simulink library "SimplusGT"  (R2024b)
settings: Solver=ode45  StartTime=0.0  StopTime=10.0  RelTol=1e-3
undefined symbols (not defined in the file or in its folder): ang_r, Cf, DiscIntNeverNeededParam, dspblkCoreblockFVToolHelper, gcbh, initial, Lc, Lf, m, OtherInputs, P_dc, Sbase, t0, Tm_pu, Ts, V, Vbase, w_droop, w_i, w_pll, w_tau, w_v, Wbase, wc, wfil, x0, Ybase, Zbase
libraries: spsVoltageMeasurementLib x107, spsCurrentMeasurementLib x92, spsControlledCurrentSourceLib x57, spsThreePhaseSeriesRLCBranchLib x29, spsControlledVoltageSourceLib x22, spsSeriesRLCBranchLib x15, SimplexPS_2015a x6, simulink x4, spsThreePhaseParallelRLCBranchLib x3, spsThreePhaseVIMeasurementLib x2, spsThreePhaseBreakerLib x2, $bdroot x1
(part 2 of 8)

== system SimplusGT/Complex2ReIm ==
  +- : Inport
  ->Im : Fcn  Expr=(u[1]-u[2])/2/1i
  ->Re : Fcn  Expr=(u[1]+u[2])/2
  Mux : Mux  Inputs=2
  Re Im : Outport
  wires:
  +-/1 -> ->Im/1, ->Re/1
  Mux/1 -> Re Im/1
  ->Re/1 -> Mux/1
  ->Im/1 -> Mux/2

== system SimplusGT/Conjugate ==
  note: Conjugate
      |
      | Author(s): Yitong Li
  In : Inport
  Complex to Real-Imag : ComplexToRealImag
  Gain : Gain  Gain=-1
  Real-Imag to Complex : RealImagToComplex
  Out : Outport
  wires:
  Complex to Real-Imag/1 -> Real-Imag to Complex/1
  Complex to Real-Imag/2 -> Gain/1
  Real-Imag to Complex/1 -> Out/1
  Gain/1 -> Real-Imag to Complex/2
  In/1 -> Complex to Real-Imag/1

== system SimplusGT/DC Infinite Bus (Current Type) ==
  note: Model for current-type dc infinite bus.
      |
      | Author(s): Yitong Li
  Bus Creator : BusCreator  Inputs=3
  Constant4 : Constant  Value=i
  Controlled Current Source : spsControlledCurrentSourceLib/Controlled Current Source  Initialize=on  Source_Type=AC  Amplitude=0  Phase=0  Frequency=0  Measurements=None
  Gain1 : Gain  Gain=1/Vbase
  Gain3 : Gain  Gain=Sbase/Vbase
  Product : Product
  RC : spsSeriesRLCBranchLib/Series RLC Branch  LConnTagsString=__new0  RConnTagsString=__new0  BranchType=RC  Resistance=R*V^2/Sbase  Inductance=1e-3  SetiL0=off  InitialCurrent=0  Capacitance=C/(2*pi*50)*Sbase/Vbase^2  Setx0=off  InitialVoltage=0  Measurements=None
  Voltage Measurement : spsVoltageMeasurementLib/Voltage Measurement  PhasorSimulation=off  OutputType=Complex  PSBequivalent=0
  + : PMIOPort  Side=Left
  - : PMIOPort  Port=2  Side=Left
  m : Outport
  wires:
  Constant4/1 -> [i], Gain3/1, Product/2
  [v] -> Bus Creator/1  "v"
  [i] -> Bus Creator/2  "i"
  Bus Creator/1 -> m/1
  Gain3/1 -> Controlled Current Source/1
  Gain1/1 -> Product/1, [v]
  [p] -> Bus Creator/3  "p"
  Product/1 -> [p]
  Voltage Measurement/1 -> Gain1/1
  connections:
  -/RConn1 -- RC/RConn1 -- Voltage Measurement/LConn2 -- Controlled Current Source/LConn1
  Controlled Current Source/RConn1 -- +/RConn1 -- RC/LConn1 -- Voltage Measurement/LConn1

== system SimplusGT/DC Infinite Bus (Voltage Type) ==
  note: Model for voltage-type dc infinite bus.
      |
      | Author(s): Yitong Li
  Bus Creator : BusCreator  Inputs=3
  Constant4 : Constant  Value=v
  Gain1 : Gain  Gain=Vbase
  Gain3 : Gain  Gain=1/(Sbase/Vbase)
  Product : Product
  R : spsSeriesRLCBranchLib/Series RLC Branch  LConnTagsString=__new0  RConnTagsString=__new0  BranchType=R  Resistance=R*Vbase^2/Sbase  Inductance=1e-3  SetiL0=off  InitialCurrent=0  Capacitance=1e-6  Setx0=off  InitialVoltage=0  Measurements=None
  i : spsCurrentMeasurementLib/Current Measurement  PhasorSimulation=off  OutputType=Complex  PSBequivalent=0
  v : spsControlledVoltageSourceLib/Controlled Voltage Source  Initialize=on  Source_Type=AC  Amplitude=0  Phase=0  Frequency=0  Measurements=None
  + : PMIOPort  Side=Left
  - : PMIOPort  Port=2  Side=Left
  m : Outport
  wires:
  Constant4/1 -> Product/2, [v], Gain1/1
  [v] -> Bus Creator/1  "v"
  [i] -> Bus Creator/2  "i"
  Bus Creator/1 -> m/1
  Gain1/1 -> v/1
  i/1 -> Gain3/1
  Gain3/1 -> Product/1, [i]
  [p] -> Bus Creator/3  "p"
  Product/1 -> [p]
  connections:
  v/LConn1 -- -/RConn1
  i/RConn1 -- v/RConn1
  R/RConn1 -- i/LConn1
  R/LConn1 -- +/RConn1

== system SimplusGT/DC Series RL Branch ==
  Branch1 : spsSeriesRLCBranchLib/Series RLC Branch  LConnTagsString=__new0  RConnTagsString=__new0  BranchType=RL  Resistance=Resistance/2  Inductance=Inductance/2  SetiL0=off  InitialCurrent=0  Capacitance=1e-6  Setx0=off  InitialVoltage=0  Measurements=None
  Branch2 : spsSeriesRLCBranchLib/Series RLC Branch  LConnTagsString=__new0  RConnTagsString=__new0  BranchType=RL  Resistance=Resistance/2  Inductance=Inductance/2  SetiL0=off  InitialCurrent=0  Capacitance=1e-6  Setx0=off  InitialVoltage=0  Measurements=None
  a+ : PMIOPort  Side=Left
  a- : PMIOPort  Port=2  Side=Right
  b+ : PMIOPort  Port=3  Side=Left
  b- : PMIOPort  Port=4  Side=Right
  connections:
  Branch1/RConn1 -- a-/RConn1
  Branch2/LConn1 -- b+/RConn1
  Branch2/RConn1 -- b-/RConn1
  Branch1/LConn1 -- a+/RConn1

== system SimplusGT/Discrete PI ==
  note: Digital PI controller
      |
      | Author(s): Yitong Li
  enable : Inport
  reference : Inport  Port=2
  initial : Inport  Port=3
  actual : Inport  Port=4
  Discrete-Time Integrator : DiscreteIntegrator  gainval=1  ExternalReset=rising  InitialConditionSource=external  InitialCondition=initial  SampleTime=Ts  LimitOutput=on  UpperSaturationLimit=xmax  LowerSaturationLimit=xmin  ICPrevOutput=DiscIntNeverNeededParam  ICPrevScaledInput=DiscIntNeverNeededParam
  Ierror : Sum  Inputs=+-
  Ki : Gain  Gain=Ki  SaturateOnIntegerOverflow=on  OutDataTypeStr=Inherit: Same as input  ParamDataTypeStr=Inherit: Same as input
  Kp : Gain  Gain=Kp  SaturateOnIntegerOverflow=on  OutDataTypeStr=Inherit: Same as input  ParamDataTypeStr=Inherit: Same as input
  Perror : Sum  Inputs=-+
  Product : Product  RndMeth=Zero
  Product1 : Product  RndMeth=Zero
  Saturation : Saturate  UpperLimit=xmax  LowerLimit=xmin
  Sum1 : Sum  SaturateOnIntegerOverflow=on
  Out : Outport
  wires:
  Saturation/1 -> Out/1
  Sum1/1 -> Saturation/1
  Ki/1 -> Discrete-Time Integrator/1
  Kp/1 -> Sum1/1
  Discrete-Time Integrator/1 -> Sum1/2
  enable/1 -> Discrete-Time Integrator/2, Product/2, Product1/2
  initial/1 -> Discrete-Time Integrator/3
  reference/1 -> Perror/2, Ierror/1
  actual/1 -> Ierror/2, Perror/1
  Perror/1 -> Product/1
  Product/1 -> Kp/1
  Ierror/1 -> Product1/1
  Product1/1 -> Ki/1

== system SimplusGT/Frequency Droop (iDQ -> id) ==
  note: Measurement
  note: Frequency droop controller
      |
      | Author(s): Yitong Li
      |
      | Notes:
      |
      | vq is fed into the PI controller of the PLL.
      |
      | This control assumes the input current is in DQ frame, which is the common electrical frame. It is not a practical frequency droop control which uses iabc or PQ as the input. But this controller is useful in research.
  iDQ : Inport
  wDQ : Inport  Port=2
  Constant : Constant  Value=w0
  Constant2 : Constant  Value=theta0
  Constant4 : Constant  Value=2*pi
  Constant6 : Constant  Value=i0
  Demux1 : Demux  Outputs=2
  Discrete-Time Integrator : DiscreteIntegrator  SampleTime=Ts  ICPrevOutput=DiscIntNeverNeededParam  ICPrevScaledInput=DiscIntNeverNeededParam
  Filter p : DiscreteTransferFcn  Numerator=w_tau*Ts  Denominator=[1 ((w_tau*Ts)-1)]  SampleTime=Ts
  Gain1 : Gain  Gain=1/(Sbase/Vbase)
  Gain2 : Gain  Gain=m
  Gain3 : Gain  Gain=Wbase
  Gain4 : Gain  Gain=1/Wbase
  Gain5 : Gain  Gain=1/pi
  Math Function1 : Math  Operator=mod  SignedPower=on
  Mux : Mux  Inputs=2
  Scope : Scope  NumInputPorts=4
  Sum : Sum
  Sum1 : Sum
  Sum2 : Sum  Inputs=+-
  Sum3 : Sum  Inputs=+-
  "x1y1 -> x2y2" : Subsystem  AncestorBlock=SimplusGT/x1y1 -> x2y2
      settings: LibrarySourceBlock=SimplusGT/x1y1 -> x2y2
  wdq : Outport
  theta : Outport  Port=2
  idq : Outport  Port=3
  wires:
  Gain1/1 -> Filter p/1
  Math Function1/1 -> "x1y1 -> x2y2"/2(theta), theta/1, [theta]
  Constant6/1 -> Sum2/1
  Constant/1 -> Sum/2
  [iq] -> Scope/2  "iq"
  Constant2/1 -> Sum1/2, [theta0]
  Constant4/1 -> Math Function1/2
  Gain2/1 -> Sum/1
  Sum1/1 -> Math Function1/1
  Discrete-Time Integrator/1 -> Sum1/1
  Gain5/1 -> Scope/4
  iDQ/1 -> "x1y1 -> x2y2"/1(x1y1)
  "x1y1 -> x2y2"/1(x2y2) -> idq/1, Demux1/1
  [theta0] -> Mux/1  "theta"
  Gain3/1 -> wdq/1, [w], Discrete-Time Integrator/1
  Sum2/1 -> Gain2/1
  Mux/1 -> Gain5/1  "theta"
  Demux1/1 -> Gain1/1, [id]  "id"
  [w] -> Gain4/1  "w"
  Gain4/1 -> Scope/3
  [theta] -> Mux/2  "theta"
  [id] -> Scope/1  "id"
  Filter p/1 -> Sum2/2
  Demux1/2 -> [iq]
  Sum/1 -> Sum3/1
  Sum3/1 -> Gain3/1
  wDQ/1 -> Sum3/2

== system SimplusGT/Frequency Droop (iabc -> id) ==
  note: Measurement
  note: id-frequency droop controller
      |
      | Author(s): Yitong Li
      |
      | Notes:
      |
      | The current reference should be in source convention.
      |
      | It is a id-frequency droop controller rather than a power-frequency droop controller.
  iabc : Inport
  Constant : Constant  Value=w0
  Constant2 : Constant  Value=theta0
  Constant4 : Constant  Value=2*pi
  Constant6 : Constant  Value=i0
  Demux1 : Demux  Outputs=2
  Discrete-Time Integrator : DiscreteIntegrator  SampleTime=Ts  ICPrevOutput=DiscIntNeverNeededParam  ICPrevScaledInput=DiscIntNeverNeededParam
  Filter p : DiscreteTransferFcn  Numerator=w_tau*Ts  Denominator=[1 ((w_tau*Ts)-1)]  SampleTime=Ts
  Gain1 : Gain  Gain=1/(Sbase/Vbase)
  Gain2 : Gain  Gain=m
  Gain3 : Gain  Gain=Wbase
  Gain4 : Gain  Gain=1/Wbase
  Gain5 : Gain  Gain=1/pi
  Math Function1 : Math  Operator=mod  SignedPower=on
  Mux : Mux  Inputs=2
  Scope : Scope  NumInputPorts=4
  Sum : Sum
  Sum1 : Sum
  Sum2 : Sum  Inputs=+-
  "abc -> dq (Power-Invariant)" : Subsystem  AncestorBlock=|
      | SimplusGT/abc -> dq
      | (Power-Invariant)
      settings: LibrarySourceBlock=|
      | SimplusGT/abc -> dq
      | (Power-Invariant)
  w : Outport
  theta : Outport  Port=2
  idq : Outport  Port=3
  wires:
  Sum1/1 -> Math Function1/1
  Constant2/1 -> Sum1/2, [theta0]
  Math Function1/1 -> "abc -> dq (Power-Invariant)"/2(theta), [theta], theta/1
  Gain2/1 -> Sum/1
  Discrete-Time Integrator/1 -> Sum1/1
  Filter p/1 -> Sum2/2
  Constant/1 -> Sum/2
  "abc -> dq (Power-Invariant)"/1(dq) -> idq/1, Demux1/1
  Constant4/1 -> Math Function1/2
  iabc/1 -> "abc -> dq (Power-Invariant)"/1(abc)
  Gain1/1 -> Filter p/1
  Constant6/1 -> Sum2/1
  Sum2/1 -> Gain2/1
  Sum/1 -> Gain3/1
  Gain3/1 -> [w], w/1, Discrete-Time Integrator/1
  Demux1/1 -> Gain1/1, [id]  "id"
  Gain5/1 -> Scope/4
  [iq] -> Scope/2  "iq"
  [theta0] -> Mux/1  "theta"
  [id] -> Scope/1  "id"
  Mux/1 -> Gain5/1  "theta"
  [theta] -> Mux/2  "theta"
  Demux1/2 -> [iq]
  [w] -> Gain4/1  "w"
  Gain4/1 -> Scope/3

== system SimplusGT/Frequency Droop (iabc -> id+jiq) ==
  note: Measurement
  note: Frame trabsformation
  note: Current-frequency droop controller
      |
      | Author(s): Yitong Li
      |
      | Notes:
      |
      | The current reference should be in source convention.
      |
      | This droop controller controls both d- and q-axis currents.
  iabc : Inport
  Constant : Constant  Value=id0
  Constant10 : Constant  Value=theta_d0
  Constant2 : Constant  Value=wd0
  Constant4 : Constant  Value=2*pi
  Constant5 : Constant  Value=wq0
  Constant8 : Constant  Value=iq0
  Constant9 : Constant  Value=theta_q0
  Demux1 : Demux  Outputs=2
  Discrete-Time Integrator : DiscreteIntegrator  SampleTime=Ts  ICPrevOutput=DiscIntNeverNeededParam  ICPrevScaledInput=DiscIntNeverNeededParam
  Discrete-Time Integrator1 : DiscreteIntegrator  SampleTime=Ts  ICPrevOutput=DiscIntNeverNeededParam  ICPrevScaledInput=DiscIntNeverNeededParam
  Exp : Math  SignedPower=on
  Filter p : DiscreteTransferFcn  Numerator=w_tau*Ts  Denominator=[1 ((w_tau*Ts)-1)]  SampleTime=Ts
  Filter p1 : DiscreteTransferFcn  Numerator=w_tau*Ts  Denominator=[1 ((w_tau*Ts)-1)]  SampleTime=Ts
  Gain : Gain  Gain=Wbase
  Gain1 : Gain  Gain=Wbase
  Gain2 : Gain  Gain=1/Wbase
  Gain4 : Gain  Gain=1/pi
  Gain5 : Gain  Gain=1/(Sbase/Vbase)
  Gain6 : Gain  Gain=m
  Gain7 : Gain  Gain=-1
  Gain8 : Gain  Gain=-1
  Gain9 : Gain  Gain=m
  Math Function1 : Math  Operator=mod  SignedPower=on
  Mux : Mux  Inputs=2
  Mux1 : Mux  Inputs=2
  Mux2 : Mux  Inputs=2
  Product : Product
  Scope : Scope  NumInputPorts=3
  Sum : Sum  Inputs=|+-
  Sum{1..2,4..5} (4 alike) : Sum
  Sum3 : Sum  Inputs=|+-
  "abc -> dq (Power-Invariant)1" : Subsystem  AncestorBlock=|
      | SimplusGT/abc -> dq
      | (Power-Invariant)
      settings: LibrarySourceBlock=|
      | SimplusGT/abc -> dq
      | (Power-Invariant)
  wd : Outport
  theta_d : Outport  Port=2
  wq : Outport  Port=3
  theta_q : Outport  Port=4
  wires:
  Gain2/1 -> Scope/2  "wdq"
  Discrete-Time Integrator/1 -> Sum5/1
  "abc -> dq (Power-Invariant)1"/1(dq) -> Gain5/1
  Math Function1/1 -> theta_d/1, [thetad]
  Mux2/1 -> Gain4/1  "thetadq"
  Constant5/1 -> Sum2/2
  Constant9/1 -> Sum4/2
  Gain5/1 -> Demux1/1
  Mux/1 -> Scope/1  "idq"
  Gain4/1 -> Scope/3  "thetadq"
  Demux1/2 -> [iq]
  Sum/1 -> Gain7/1
  Constant4/1 -> Math Function1/2
  Sum4/1 -> theta_q/1, [thetaq]
  Demux1/1 -> [id]
  Sum5/1 -> Math Function1/1
  Constant8/1 -> Sum3/2
  [wd] -> Mux1/1
  Constant/1 -> Sum/2
  [iq] -> Mux/2
  [thetaq] -> Mux2/2
  Mux1/1 -> Gain2/1  "wdq"
  Exp/1 -> Product/2
  [thetad] -> Mux2/1
  Constant2/1 -> Sum1/2
  [thetaq] -> Exp/1
  Constant10/1 -> Sum5/2
  [id] -> Mux/1
  Product/1 -> "abc -> dq (Power-Invariant)1"/1(abc)
  Discrete-Time Integrator1/1 -> Sum4/1
  Filter p/1 -> Sum3/1
  [thetad] -> "abc -> dq (Power-Invariant)1"/2(theta)
  [id] -> Filter p1/1
  iabc/1 -> Product/1
  [wq] -> Mux1/2
  [iq] -> Filter p/1
  Filter p1/1 -> Sum/1
  Gain9/1 -> Sum2/1
  Gain6/1 -> Sum1/1
  Gain7/1 -> Gain6/1
  Sum3/1 -> Gain8/1
  Gain8/1 -> Gain9/1
  Gain/1 -> [wd], wd/1, Discrete-Time Integrator/1
  Sum1/1 -> Gain/1
  Sum2/1 -> Gain1/1
  Gain1/1 -> [wq], wq/1, Discrete-Time Integrator1/1

== system SimplusGT/Frequency Droop (iabc -> iq) ==
  note: iq-frequency droop controller
      |
      | Author(s): Yitong Li
      |
      | Notes:
      |
      | The current reference should be in source convention.
      |
      | It is a iq-frequency droop controller rather than a power-frequency droop controller.
  note: Measurement
  iabc : Inport
  Constant : Constant  Value=w0
  Constant2 : Constant  Value=theta0
  Constant4 : Constant  Value=2*pi
  Constant6 : Constant  Value=i0
  Demux1 : Demux  Outputs=2
  Discrete-Time Integrator : DiscreteIntegrator  SampleTime=Ts  ICPrevOutput=DiscIntNeverNeededParam  ICPrevScaledInput=DiscIntNeverNeededParam
  Filter p : DiscreteTransferFcn  Numerator=w_tau*Ts  Denominator=[1 ((w_tau*Ts)-1)]  SampleTime=Ts
  Gain1 : Gain  Gain=1/(Sbase/Vbase)
  Gain2 : Gain  Gain=m
  Gain3 : Gain  Gain=Wbase
  Gain4 : Gain  Gain=1/Wbase
  Gain5 : Gain  Gain=1/pi
  Math Function1 : Math  Operator=mod  SignedPower=on
  Mux : Mux  Inputs=2
  Scope : Scope  NumInputPorts=4
  Sum : Sum
  Sum1 : Sum
  Sum2 : Sum  Inputs=+-
  "abc -> dq (Power-Invariant)1" : Subsystem  AncestorBlock=|
      | SimplusGT/abc -> dq
      | (Power-Invariant)
      settings: LibrarySourceBlock=|
      | SimplusGT/abc -> dq
      | (Power-Invariant)
  w : Outport
  theta : Outport  Port=2
  idq : Outport  Port=3
  wires:
  Demux1/2 -> Gain1/1, [iq]
  Sum1/1 -> Math Function1/1
  Gain3/1 -> Discrete-Time Integrator/1, [w], w/1
  Filter p/1 -> Sum2/2
  Constant6/1 -> Sum2/1
  Gain1/1 -> Filter p/1
  Discrete-Time Integrator/1 -> Sum1/1
  Constant2/1 -> [theta0], Sum1/2
  Sum2/1 -> Gain2/1
  Sum/1 -> Gain3/1
  Constant/1 -> Sum/2
  "abc -> dq (Power-Invariant)1"/1(dq) -> idq/1, Demux1/1
  Constant4/1 -> Math Function1/2
  Math Function1/1 -> [theta], theta/1, "abc -> dq (Power-Invariant)1"/2(theta)
  Gain2/1 -> Sum/1
  iabc/1 -> "abc -> dq (Power-Invariant)1"/1(abc)
  [iq] -> Scope/2  "iq"
  Mux/1 -> Gain5/1
  [theta0] -> Mux/1  "theta"
  [id] -> Scope/1  "id"
  Gain5/1 -> Scope/4
  [theta] -> Mux/2  "theta"
  Demux1/1 -> [id]  "id"
  Gain4/1 -> Scope/3
  [w] -> Gain4/1  "w"

== system SimplusGT/Grid-Feeding Buck (System Object) ==
  note: Matlab System Object
  note: Auxiliary
  note: Electrical Circuit
  note: Grid-feeding buck dc-dc converter.
      |
      | Author(s): Yitong Li
      |
      | Notes:
      |
      | The model is based on matlab system object.
      |
      | The model is in load convention.
  Bus Creator : BusCreator  Inputs=4
  Constant : Constant  Value=OtherInputs
  Current Measurement : spsCurrentMeasurementLib/Current Measurement  PhasorSimulation=off  OutputType=Complex  PSBequivalent=0
  Demux : Demux  Outputs=2
  Gain1 : Gain  Gain=1/Vbase
  Gain2 : Gain  Gain=Sbase/Vbase
  Gain3 : Gain  Gain=1/(Sbase/Vbase)
  MATLAB System1 : MATLABSystem  System=SimplusGT.Class.GridFeedingBuck  Ts=Ts  Para=ApparatusPara  ApparatusType=ApparatusType  PowerFlow=PowerFlow  x0=x0  DiscreMethod=DiscreMethod  LinearizationTimes=LinearizationTimes  DirectFeedthrough=DirectFeedthrough  VirtualResistor=DiscreDampingFlag  EquiInitial=true  ElecPortIOs=[1]  SimulateUsing=Code generation
      mask Type: SimplusGT.Class.GridFeedingBuck
      mask Display:
      | disp('GridFeedingBuck');
      | port_label('input',1,'u');
      | port_label('output',1,'y');
  Mux2 : Mux  Inputs=2
  Product : Product
  R_VD : spsSeriesRLCBranchLib/Series RLC Branch  LConnTagsString=__new0  RConnTagsString=__new0  BranchType=R  Resistance=DiscreDampingValue*Vbase^2/Sbase  Inductance=1e-3  SetiL0=off  InitialCurrent=0  Capacitance=1e-6  Setx0=off  InitialVoltage=0  Measurements=None
  ia : spsControlledCurrentSourceLib/Controlled Current Source  Initialize=on  Source_Type=AC  Amplitude=0  Phase=0  Frequency=0  Measurements=None
  v : spsVoltageMeasurementLib/Voltage Measurement  PhasorSimulation=off  OutputType=Complex  PSBequivalent=0
  a : PMIOPort  Side=Left
  b : PMIOPort  Port=2  Side=Left
  m : Outport
  wires:
  Gain2/1 -> ia/1
  v/1 -> Gain1/1
  [v] -> Mux2/1
  [v] -> Bus Creator/1  "v"
  Gain1/1 -> [v]
  Demux/1 -> [i]
  Mux2/1 -> MATLAB System1/1
  MATLAB System1/1 -> Demux/1
  Demux/2 -> [v_dc]
  Bus Creator/1 -> m/1
  [i] -> Gain2/1
  Product/1 -> [p]
  Constant/1 -> Mux2/2
  [v] -> Product/1  "v"
  [i_t] -> Product/2  "i"
  [i_t] -> Bus Creator/2  "i"
  [p] -> Bus Creator/3  "p"
  [v_dc] -> Bus Creator/4  "v_dc"
  Current Measurement/1 -> Gain3/1
  Gain3/1 -> [i_t]
  connections:
  b/RConn1 -- v/LConn2 -- ia/RConn1 -- R_VD/RConn1
  R_VD/LConn1 -- Current Measurement/RConn1 -- v/LConn1 -- ia/LConn1
  Current Measurement/LConn1 -- a/RConn1

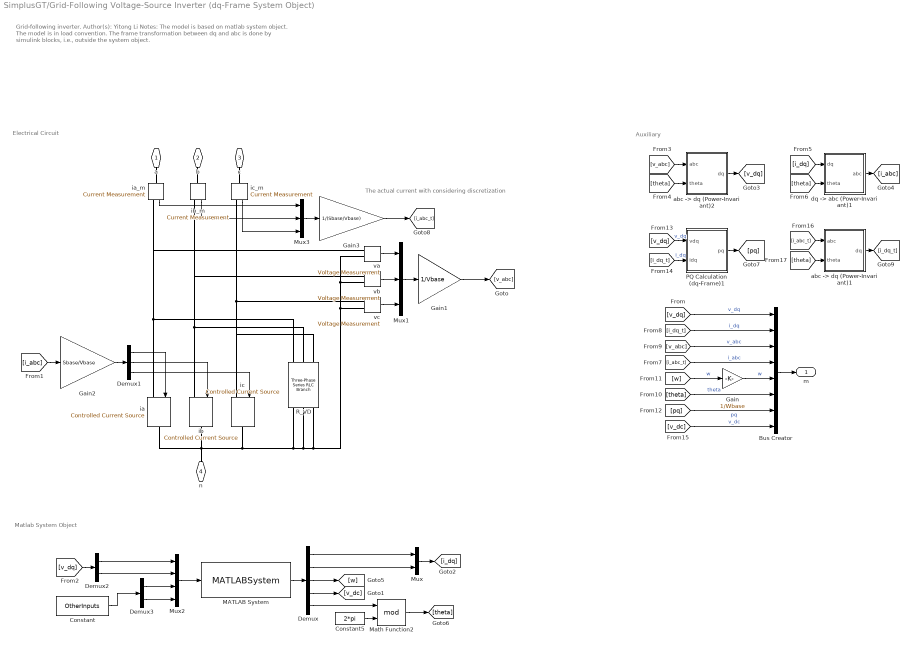
== system SimplusGT/Grid-Following Voltage-Source Inverter (dq-Frame System Object) ==
  note: Matlab System Object
  note: Auxiliary
  note: Electrical Circuit
  note: Grid-following inverter.
      |
      | Author(s): Yitong Li
      |
      | Notes:
      |
      | The model is based on matlab system object.
      |
      | The model is in load convention.
      |
      | The frame transformation between dq and abc is done by simulink blocks, i.e., outside the system object.
  note: The actual current with considering discretization
  Bus Creator : BusCreator  Inputs=8
  Constant : Constant  Value=OtherInputs
  Constant5 : Constant  Value=2*pi
  Demux : Demux  Outputs=5
  Demux1 : Demux  Outputs=3
  Demux2 : Demux  Outputs=2
  Demux3 : Demux  Outputs=2
  Gain : Gain  Gain=1/Wbase
  Gain1 : Gain  Gain=1/Vbase
  Gain2 : Gain  Gain=Sbase/Vbase
  Gain3 : Gain  Gain=1/(Sbase/Vbase)
  MATLAB System : MATLABSystem  System=SimplusGT.Class.GridFollowingVSI  Ts=Ts  Para=ApparatusPara  ApparatusType=ApparatusType  PowerFlow=PowerFlow  x0=x0  DiscreMethod=DiscreMethod  LinearizationTimes=LinearizationTimes  DirectFeedthrough=DirectFeedthrough  VirtualResistor=DiscreDampingFlag  EquiInitial=true  ElecPortIOs=[ 1, 2 ]  SimulateUsing=Code generation
      mask Type: SimplusGT.Class.GridFollowingVSI
      mask Display:
      | disp('GridFollowingVSI');
      | port_label('input',1,'u');
      | port_label('output',1,'y');
  Math Function2 : Math  Operator=mod  SignedPower=on
  Mux : Mux  Inputs=2
  Mux1 : Mux  Inputs=3
  Mux2 : Mux
  Mux3 : Mux  Inputs=3
  PQ Calculation (dq-Frame)1 : Subsystem  AncestorBlock=|
      | SimplusGT/PQ Calculation
      | (dq-Frame)
      settings: LibrarySourceBlock=|
      | SimplusGT/PQ Calculation
      | (dq-Frame)
  R_VD : spsThreePhaseSeriesRLCBranchLib/Three-Phase Series RLC Branch  LConnTagsString=A|B|C  RConnTagsString=A|B|C  BranchType=R  Resistance=DiscreDampingValue*Vbase^2/Sbase  Inductance=1e-3  Capacitance=1e-6  Measurements=None
  "abc -> dq (Power-Invariant)1" : Subsystem  AncestorBlock=|
      | SimplusGT/abc -> dq
      | (Power-Invariant)
      settings: LibrarySourceBlock=|
      | SimplusGT/abc -> dq
      | (Power-Invariant)
  "abc -> dq (Power-Invariant)2" : Subsystem  AncestorBlock=|
      | SimplusGT/abc -> dq
      | (Power-Invariant)
      settings: LibrarySourceBlock=|
      | SimplusGT/abc -> dq
      | (Power-Invariant)
  "dq -> abc (Power-Invariant)1" : Subsystem  AncestorBlock=|
      | SimplusGT/dq -> abc
      | (Power-Invariant)
      settings: LibrarySourceBlock=|
      | SimplusGT/dq -> abc
      | (Power-Invariant)
  ia : spsControlledCurrentSourceLib/Controlled Current Source  Initialize=on  Source_Type=AC  Amplitude=0  Phase=0  Frequency=0  Measurements=None
  ia_m : spsCurrentMeasurementLib/Current Measurement  PhasorSimulation=off  OutputType=Complex  PSBequivalent=0
  ib : spsControlledCurrentSourceLib/Controlled Current Source  Initialize=on  Source_Type=AC  Amplitude=0  Phase=0  Frequency=0  Measurements=None
  ib_m : spsCurrentMeasurementLib/Current Measurement  PhasorSimulation=off  OutputType=Complex  PSBequivalent=0
  ic : spsControlledCurrentSourceLib/Controlled Current Source  Initialize=on  Source_Type=AC  Amplitude=0  Phase=0  Frequency=0  Measurements=None
  ic_m : spsCurrentMeasurementLib/Current Measurement  PhasorSimulation=off  OutputType=Complex  PSBequivalent=0
  va : spsVoltageMeasurementLib/Voltage Measurement  PhasorSimulation=off  OutputType=Complex  PSBequivalent=0
  vb : spsVoltageMeasurementLib/Voltage Measurement  PhasorSimulation=off  OutputType=Complex  PSBequivalent=0
  vc : spsVoltageMeasurementLib/Voltage Measurement  PhasorSimulation=off  OutputType=Complex  PSBequivalent=0
  a : PMIOPort  Side=Left
  b : PMIOPort  Port=2  Side=Left
  c : PMIOPort  Port=3  Side=Left
  n : PMIOPort  Port=4  Side=Left
  m : Outport
  wires:
  Demux/2 -> Mux/2
  Demux/1 -> Mux/1
  Mux/1 -> [i_dq]
  Demux/3 -> [w]
  Demux1/1 -> ia/1
  Demux1/2 -> ib/1
  va/1 -> Mux1/1
  vb/1 -> Mux1/2
  Mux1/1 -> Gain1/1
  [v_dq] -> Demux2/1
  Demux2/1 -> Mux2/1
  Demux2/2 -> Mux2/2
  [v_dq] -> Bus Creator/1  "v_dq"
  [i_dq_t] -> Bus Creator/2  "i_dq"
  [v_abc] -> Bus Creator/3  "v_abc"
  [i_abc_t] -> Bus Creator/4  "i_abc"
  [theta] -> Bus Creator/6  "theta"
  [v_abc] -> "abc -> dq (Power-Invariant)2"/1(abc)
  [theta] -> "abc -> dq (Power-Invariant)2"/2(theta)
  "abc -> dq (Power-Invariant)2"/1(dq) -> [v_dq]
  [i_dq] -> "dq -> abc (Power-Invariant)1"/1(dq)
  [theta] -> "dq -> abc (Power-Invariant)1"/2(theta)
  "dq -> abc (Power-Invariant)1"/1(abc) -> [i_abc]
  Mux2/1 -> MATLAB System/1
  MATLAB System/1 -> Demux/1
  vc/1 -> Mux1/3
  Demux1/3 -> ic/1
  Demux/5 -> Math Function2/1
  Constant5/1 -> Math Function2/2
  Math Function2/1 -> [theta]
  Demux/4 -> [v_dc]
  Bus Creator/1 -> m/1
  Demux3/1 -> Mux2/3
  Demux3/2 -> Mux2/4
  Constant/1 -> Demux3/1
  [w] -> Gain/1  "w"
  Gain/1 -> Bus Creator/5  "w"
  [i_abc] -> Gain2/1
  [pq] -> Bus Creator/7  "pq"
  [v_dq] -> PQ Calculation (dq-Frame)1/1(vdq)  "v_dq"
  [i_dq_t] -> PQ Calculation (dq-Frame)1/2(idq)  "i_dq"
  PQ Calculation (dq-Frame)1/1(pq) -> [pq]
  Gain2/1 -> Demux1/1
  Gain1/1 -> [v_abc]
  [v_dc] -> Bus Creator/8  "v_dc"
  ic_m/1 -> Mux3/3
  Gain3/1 -> [i_abc_t]
  Mux3/1 -> Gain3/1
  ib_m/1 -> Mux3/2
  ia_m/1 -> Mux3/1
  [theta] -> "abc -> dq (Power-Invariant)1"/2(theta)
  [i_abc_t] -> "abc -> dq (Power-Invariant)1"/1(abc)
  "abc -> dq (Power-Invariant)1"/1(dq) -> [i_dq_t]
  connections:
  vb/LConn2 -- va/LConn2 -- vc/LConn2 -- R_VD/RConn3 -- R_VD/RConn2 -- R_VD/RConn1 -- ic/RConn1 -- ia/RConn1 -- ib/RConn1 -- n/RConn1
  R_VD/LConn1 -- va/LConn1 -- ia_m/RConn1 -- ia/LConn1
  R_VD/LConn2 -- ib_m/RConn1 -- vb/LConn1 -- ib/LConn1
  R_VD/LConn3 -- ic/LConn1 -- ic_m/RConn1 -- vc/LConn1
  ic_m/LConn1 -- c/RConn1
  ib_m/LConn1 -- b/RConn1
  ia_m/LConn1 -- a/RConn1

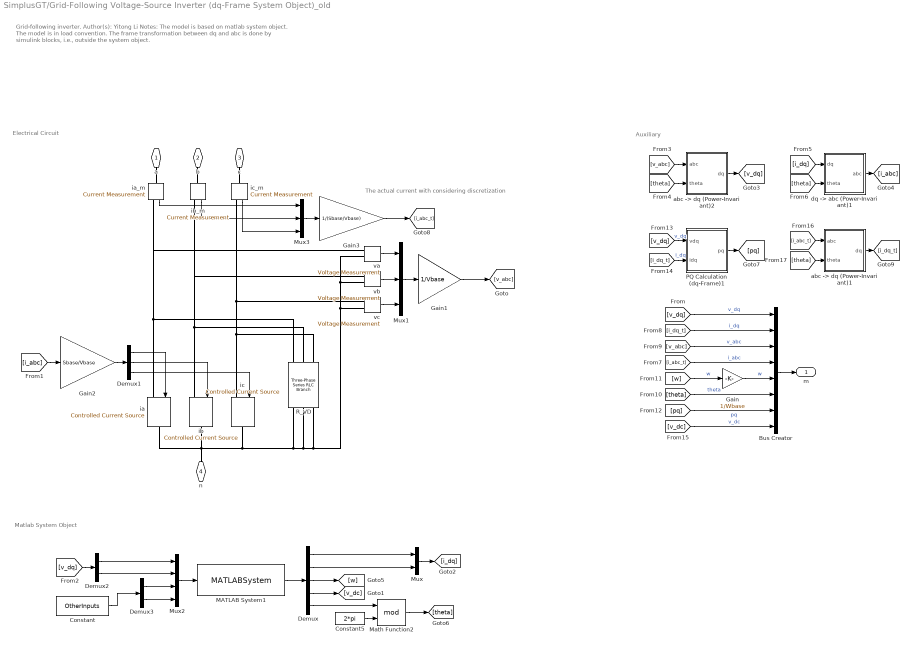
== system SimplusGT/Grid-Following Voltage-Source Inverter (dq-Frame System Object)_old ==
  note: Matlab System Object
  note: Auxiliary
  note: Electrical Circuit
  note: Grid-following inverter.
      |
      | Author(s): Yitong Li
      |
      | Notes:
      |
      | The model is based on matlab system object.
      |
      | The model is in load convention.
      |
      | The frame transformation between dq and abc is done by simulink blocks, i.e., outside the system object.
  note: The actual current with considering discretization
  Bus Creator : BusCreator  Inputs=8
  Constant : Constant  Value=OtherInputs
  Constant5 : Constant  Value=2*pi
  Demux : Demux  Outputs=5
  Demux1 : Demux  Outputs=3
  Demux2 : Demux  Outputs=2
  Demux3 : Demux  Outputs=2
  Gain : Gain  Gain=1/Wbase
  Gain1 : Gain  Gain=1/Vbase
  Gain2 : Gain  Gain=Sbase/Vbase
  Gain3 : Gain  Gain=1/(Sbase/Vbase)
  MATLAB System1 : MATLABSystem  System=SimplusGT.Class.GridFollowingVSI_old  Ts=Ts  Para=ApparatusPara  ApparatusType=ApparatusType  PowerFlow=PowerFlow  x0=x0  DiscreMethod=DiscreMethod  LinearizationTimes=LinearizationTimes  DirectFeedthrough=DirectFeedthrough  VirtualResistor=DiscreDampingFlag  EquiInitial=true  ElecPortIOs=[ 1, 2 ]  SimulateUsing=Code generation
      mask Type: SimplusGT.Class.GridFollowingVSI_old
      mask Display:
      | disp('GridFollowingVSI_old');
      | port_label('input',1,'u');
      | port_label('output',1,'y');
  Math Function2 : Math  Operator=mod  SignedPower=on
  Mux : Mux  Inputs=2
  Mux1 : Mux  Inputs=3
  Mux2 : Mux
  Mux3 : Mux  Inputs=3
  PQ Calculation (dq-Frame)1 : Subsystem  AncestorBlock=|
      | SimplusGT/PQ Calculation
      | (dq-Frame)
      settings: LibrarySourceBlock=|
      | SimplusGT/PQ Calculation
      | (dq-Frame)
  R_VD : spsThreePhaseSeriesRLCBranchLib/Three-Phase Series RLC Branch  LConnTagsString=A|B|C  RConnTagsString=A|B|C  BranchType=R  Resistance=DiscreDampingValue*Vbase^2/Sbase  Inductance=1e-3  Capacitance=1e-6  Measurements=None
  "abc -> dq (Power-Invariant)1" : Subsystem  AncestorBlock=|
      | SimplusGT/abc -> dq
      | (Power-Invariant)
      settings: LibrarySourceBlock=|
      | SimplusGT/abc -> dq
      | (Power-Invariant)
  "abc -> dq (Power-Invariant)2" : Subsystem  AncestorBlock=|
      | SimplusGT/abc -> dq
      | (Power-Invariant)
      settings: LibrarySourceBlock=|
      | SimplusGT/abc -> dq
      | (Power-Invariant)
  "dq -> abc (Power-Invariant)1" : Subsystem  AncestorBlock=|
      | SimplusGT/dq -> abc
      | (Power-Invariant)
      settings: LibrarySourceBlock=|
      | SimplusGT/dq -> abc
      | (Power-Invariant)
  ia : spsControlledCurrentSourceLib/Controlled Current Source  Initialize=on  Source_Type=AC  Amplitude=0  Phase=0  Frequency=0  Measurements=None
  ia_m : spsCurrentMeasurementLib/Current Measurement  PhasorSimulation=off  OutputType=Complex  PSBequivalent=0
  ib : spsControlledCurrentSourceLib/Controlled Current Source  Initialize=on  Source_Type=AC  Amplitude=0  Phase=0  Frequency=0  Measurements=None
  ib_m : spsCurrentMeasurementLib/Current Measurement  PhasorSimulation=off  OutputType=Complex  PSBequivalent=0
  ic : spsControlledCurrentSourceLib/Controlled Current Source  Initialize=on  Source_Type=AC  Amplitude=0  Phase=0  Frequency=0  Measurements=None
  ic_m : spsCurrentMeasurementLib/Current Measurement  PhasorSimulation=off  OutputType=Complex  PSBequivalent=0
  va : spsVoltageMeasurementLib/Voltage Measurement  PhasorSimulation=off  OutputType=Complex  PSBequivalent=0
  vb : spsVoltageMeasurementLib/Voltage Measurement  PhasorSimulation=off  OutputType=Complex  PSBequivalent=0
  vc : spsVoltageMeasurementLib/Voltage Measurement  PhasorSimulation=off  OutputType=Complex  PSBequivalent=0
  a : PMIOPort  Side=Left
  b : PMIOPort  Port=2  Side=Left
  c : PMIOPort  Port=3  Side=Left
  n : PMIOPort  Port=4  Side=Left
  m : Outport
  wires:
  Demux/2 -> Mux/2
  Demux/1 -> Mux/1
  Mux/1 -> [i_dq]
  Demux/3 -> [w]
  Demux1/1 -> ia/1
  Demux1/2 -> ib/1
  va/1 -> Mux1/1
  vb/1 -> Mux1/2
  Mux1/1 -> Gain1/1
  [v_dq] -> Demux2/1
  Demux2/1 -> Mux2/1
  Demux2/2 -> Mux2/2
  [v_dq] -> Bus Creator/1  "v_dq"
  [i_dq_t] -> Bus Creator/2  "i_dq"
  [v_abc] -> Bus Creator/3  "v_abc"
  [i_abc_t] -> Bus Creator/4  "i_abc"
  [theta] -> Bus Creator/6  "theta"
  [v_abc] -> "abc -> dq (Power-Invariant)2"/1(abc)
  [theta] -> "abc -> dq (Power-Invariant)2"/2(theta)
  "abc -> dq (Power-Invariant)2"/1(dq) -> [v_dq]
  [i_dq] -> "dq -> abc (Power-Invariant)1"/1(dq)
  [theta] -> "dq -> abc (Power-Invariant)1"/2(theta)
  "dq -> abc (Power-Invariant)1"/1(abc) -> [i_abc]
  Mux2/1 -> MATLAB System1/1
  MATLAB System1/1 -> Demux/1
  vc/1 -> Mux1/3
  Demux1/3 -> ic/1
  Demux/5 -> Math Function2/1
  Constant5/1 -> Math Function2/2
  Math Function2/1 -> [theta]
  Demux/4 -> [v_dc]
  Bus Creator/1 -> m/1
  Demux3/1 -> Mux2/3
  Demux3/2 -> Mux2/4
  Constant/1 -> Demux3/1
  [w] -> Gain/1  "w"
  Gain/1 -> Bus Creator/5  "w"
  [i_abc] -> Gain2/1
  [pq] -> Bus Creator/7  "pq"
  [v_dq] -> PQ Calculation (dq-Frame)1/1(vdq)  "v_dq"
  [i_dq_t] -> PQ Calculation (dq-Frame)1/2(idq)  "i_dq"
  PQ Calculation (dq-Frame)1/1(pq) -> [pq]
  Gain2/1 -> Demux1/1
  Gain1/1 -> [v_abc]
  [v_dc] -> Bus Creator/8  "v_dc"
  ic_m/1 -> Mux3/3
  Gain3/1 -> [i_abc_t]
  Mux3/1 -> Gain3/1
  ib_m/1 -> Mux3/2
  ia_m/1 -> Mux3/1
  [theta] -> "abc -> dq (Power-Invariant)1"/2(theta)
  [i_abc_t] -> "abc -> dq (Power-Invariant)1"/1(abc)
  "abc -> dq (Power-Invariant)1"/1(dq) -> [i_dq_t]
  connections:
  vb/LConn2 -- va/LConn2 -- vc/LConn2 -- R_VD/RConn3 -- R_VD/RConn2 -- R_VD/RConn1 -- ic/RConn1 -- ia/RConn1 -- ib/RConn1 -- n/RConn1
  R_VD/LConn1 -- va/LConn1 -- ia_m/RConn1 -- ia/LConn1
  R_VD/LConn2 -- ib_m/RConn1 -- vb/LConn1 -- ib/LConn1
  R_VD/LConn3 -- ic/LConn1 -- ic_m/RConn1 -- vc/LConn1
  ic_m/LConn1 -- c/RConn1
  ib_m/LConn1 -- b/RConn1
  ia_m/LConn1 -- a/RConn1

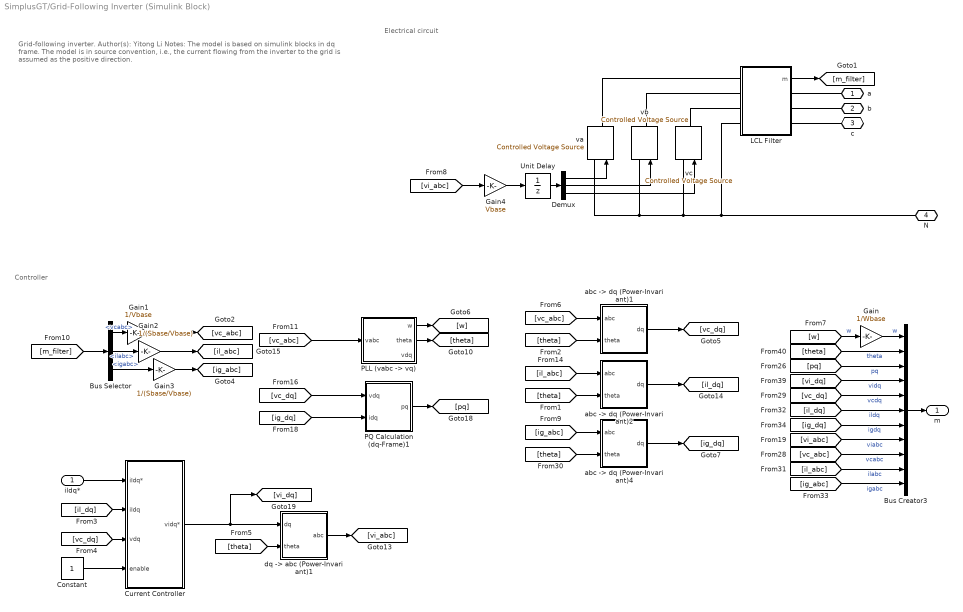
== system SimplusGT/Grid-Following Inverter (Simulink Block) ==
  note: Controller
  note: Electrical circuit
  note: Grid-following inverter.
      |
      | Author(s): Yitong Li
      |
      | Notes:
      |
      | The model is based on simulink blocks in dq frame.
      |
      | The model is in source convention, i.e., the current flowing from the inverter to the grid is assumed as the positive direction.
  ildq* : Inport
  Bus Creator3 : BusCreator  Inputs=11
  Bus Selector : BusSelector  OutputSignals=vcabc,ilabc,igabc
  Constant : Constant
  Current Controller : Subsystem  mask{Ts=Ts, Wbase=Wbase, Lf=Lf*(Vbase^2/Sbase)/Wbase, Kg=0, Kp=w_i*Lf*(Vbase^2/Sbase)/Wbase, Ki=w_i*w_i/4*Lf*(Vbase^2/Sbase)/Wbase, vdmax=inf, vqmax=inf, Kcd=0}
      mask prompts: Ts "Sampling Time (s)"; Wbase "Base Angular Frequency (rad/s)"; Lf "Inductance"; Kg "Estimator Gain"; Kp "Proportional Gain"; Ki "Integral Gain"; vdmax "Voltage D Limit"; vqmax "Voltage Q Limit"; Kcd "Cross Decoupling Gain"
  Demux : Demux  Outputs=3
  Gain : Gain  Gain=1/Wbase
  Gain1 : Gain  Gain=1/Vbase
  Gain2 : Gain  Gain=1/(Sbase/Vbase)
  Gain3 : Gain  Gain=1/(Sbase/Vbase)
  Gain4 : Gain  Gain=Vbase
  LCL Filter : Subsystem  AncestorBlock=SimplexPS/LCL Filter  mask{Lf=Lf*Zbase/Wbase, Rf=1e-9, Lc=Lc*(Vbase^2/Sbase)/Wbase, Rc=1e-9, Cf=Cf*(Sbase/Vbase^2)/Wbase, Rd=1e-20}
      mask prompts: Lf "Lf (H)"; Rf "Rf (Ohm)"; Lc "Lc (H)"; Rc "Rc (Ohm)"; Cf "Cf (F)"; Rd "Rd (Ohm)"
      settings: LibrarySourceBlock=SimplexPS/LCL Filter
  "PLL (vabc -> vq)" : Subsystem  AncestorBlock=|  mask{Ts=Ts, Vbase=Vbase, Wbase=Wbase, w_pll=w_pll, w_tau=w_tau, theta0=0}
      | SimplusGT/PLL
      | (vabc -> vq)
      mask prompts: Ts "Ts (s), sampling period"; Vbase "Vbase (V), base voltage"; Wbase "Wbase (rad/s), base angular frequency"; w_pll "w_pll (rad/s), PLL bandwidth"; w_tau "w_tau (rad/s), low-pass filter bandwidth"; theta0 "theta0 (rad), initial angle"
      settings: LibrarySourceBlock=|
      | SimplusGT/PLL
      | (vabc -> vq)
  PQ Calculation (dq-Frame)1 : Subsystem  AncestorBlock=|
      | SimplusGT/PQ Calculation
      | (dq-Frame)
      settings: LibrarySourceBlock=|
      | SimplusGT/PQ Calculation
      | (dq-Frame)
  Unit Delay : UnitDelay  SampleTime=-1  HasFrameUpgradeWarning=on
  "abc -> dq (Power-Invariant)1" : Subsystem  AncestorBlock=|
      | SimplusGT/abc -> dq
      | (Power-Invariant)
      settings: LibrarySourceBlock=|
      | SimplusGT/abc -> dq
      | (Power-Invariant)
  "abc -> dq (Power-Invariant)2" : Subsystem  AncestorBlock=|
      | SimplusGT/abc -> dq
      | (Power-Invariant)
      settings: LibrarySourceBlock=|
      | SimplusGT/abc -> dq
      | (Power-Invariant)
  "abc -> dq (Power-Invariant)4" : Subsystem  AncestorBlock=|
      | SimplusGT/abc -> dq
      | (Power-Invariant)
      settings: LibrarySourceBlock=|
      | SimplusGT/abc -> dq
      | (Power-Invariant)
  "dq -> abc (Power-Invariant)1" : Subsystem  AncestorBlock=|
      | SimplusGT/dq -> abc
      | (Power-Invariant)
      settings: LibrarySourceBlock=|
      | SimplusGT/dq -> abc
      | (Power-Invariant)
  va : spsControlledVoltageSourceLib/Controlled Voltage Source  Initialize=on  Source_Type=AC  Amplitude=0  Phase=0  Frequency=0  Measurements=None
  vb : spsControlledVoltageSourceLib/Controlled Voltage Source  Initialize=on  Source_Type=AC  Amplitude=0  Phase=0  Frequency=0  Measurements=None
  vc : spsControlledVoltageSourceLib/Controlled Voltage Source  Initialize=on  Source_Type=AC  Amplitude=0  Phase=0  Frequency=0  Measurements=None
  a : PMIOPort  Side=Right
  b : PMIOPort  Port=2  Side=Right
  c : PMIOPort  Port=3  Side=Right
  N : PMIOPort  Port=4  Side=Right
  m : Outport
  wires:
  "dq -> abc (Power-Invariant)1"/1(abc) -> [vi_abc]
  Bus Creator3/1 -> m/1
  LCL Filter/1(m) -> [m_filter]
  Demux/1 -> va/1
  Demux/2 -> vb/1
  Demux/3 -> vc/1
  [theta] -> "abc -> dq (Power-Invariant)1"/2(theta)
  [theta] -> "abc -> dq (Power-Invariant)2"/2(theta)
  [vc_abc] -> "abc -> dq (Power-Invariant)1"/1(abc)
  [il_abc] -> "abc -> dq (Power-Invariant)2"/1(abc)
  [ig_abc] -> "abc -> dq (Power-Invariant)4"/1(abc)
  [theta] -> "abc -> dq (Power-Invariant)4"/2(theta)
  Bus Selector/3 -> Gain3/1  "<igabc>"
  Bus Selector/2 -> Gain2/1  "<ilabc>"
  "PLL (vabc -> vq)"/2(theta) -> [theta]
  "PLL (vabc -> vq)"/1(w) -> [w]
  Constant/1 -> Current Controller/4(enable)
  [vc_dq] -> Current Controller/3(vdq)
  Current Controller/1(vidq*) -> "dq -> abc (Power-Invariant)1"/1(dq), [vi_dq]
  [theta] -> "dq -> abc (Power-Invariant)1"/2(theta)
  [vc_dq] -> PQ Calculation (dq-Frame)1/1(vdq)
  PQ Calculation (dq-Frame)1/1(pq) -> [pq]
  [ig_dq] -> PQ Calculation (dq-Frame)1/2(idq)
  ildq*/1 -> Current Controller/1(iIdq*)
  [il_dq] -> Current Controller/2(iIdq)
  [vc_abc] -> "PLL (vabc -> vq)"/1(vabc)
  "abc -> dq (Power-Invariant)1"/1(dq) -> [vc_dq]
  "abc -> dq (Power-Invariant)4"/1(dq) -> [ig_dq]
  "abc -> dq (Power-Invariant)2"/1(dq) -> [il_dq]
  [m_filter] -> Bus Selector/1
  Unit Delay/1 -> Demux/1
  Bus Selector/1 -> Gain1/1  "<vcabc>"
  [w] -> Gain/1  "w"
  Gain/1 -> Bus Creator3/1  "w"
  [theta] -> Bus Creator3/2  "theta"
  [pq] -> Bus Creator3/3  "pq"
  [vi_dq] -> Bus Creator3/4  "vidq"
  [vc_dq] -> Bus Creator3/5  "vcdq"
  [il_dq] -> Bus Creator3/6  "ildq"
  [ig_dq] -> Bus Creator3/7  "igdq"
  [vi_abc] -> Bus Creator3/8  "viabc"
  [vc_abc] -> Bus Creator3/9  "vcabc"
  [il_abc] -> Bus Creator3/10  "ilabc"
  [ig_abc] -> Bus Creator3/11  "igabc"
  Gain1/1 -> [vc_abc]
  Gain2/1 -> [il_abc]
  Gain3/1 -> [ig_abc]
  Gain4/1 -> Unit Delay/1
  [vi_abc] -> Gain4/1
  connections:
  LCL Filter/LConn2 -- vb/RConn1
  LCL Filter/LConn1 -- va/RConn1
  LCL Filter/RConn1 -- a/RConn1
  LCL Filter/RConn2 -- b/RConn1
  LCL Filter/RConn3 -- c/RConn1
  N/RConn1 -- LCL Filter/LConn4 -- vc/LConn1 -- vb/LConn1 -- va/LConn1
  LCL Filter/LConn3 -- vc/RConn1

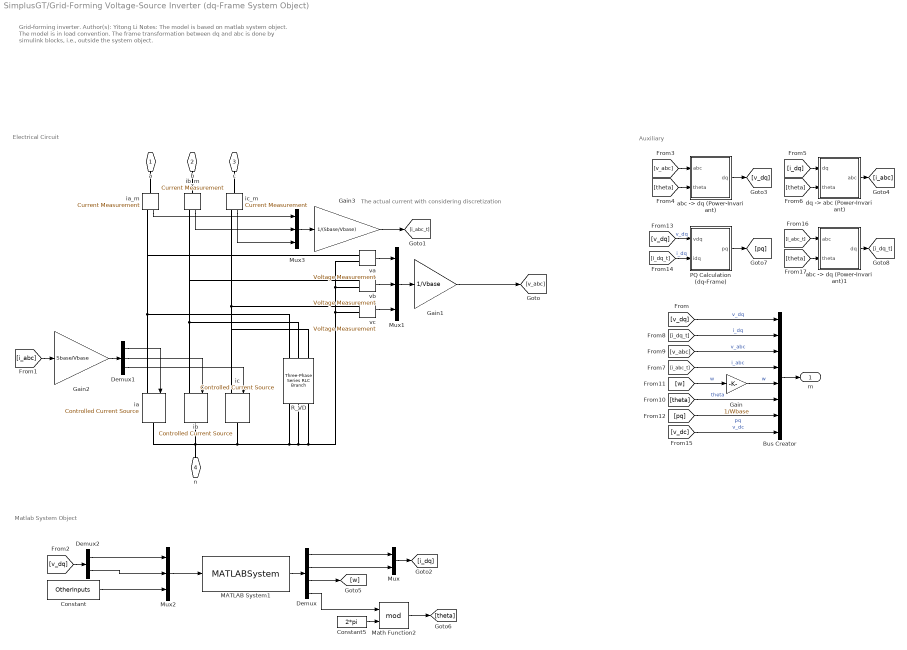
== system SimplusGT/Grid-Forming Voltage-Source Inverter (dq-Frame System Object) ==
  note: Matlab System Object
  note: Auxiliary
  note: Electrical Circuit
  note: Grid-forming inverter.
      |
      | Author(s): Yitong Li
      |
      | Notes:
      |
      | The model is based on matlab system object.
      |
      | The model is in load convention.
      |
      | The frame transformation between dq and abc is done by simulink blocks, i.e., outside the system object.
  note: The actual current with considering discretization
  Bus Creator : BusCreator  Inputs=8
  Constant : Constant  Value=OtherInputs
  Constant5 : Constant  Value=2*pi
  Demux : Demux
  Demux1 : Demux  Outputs=3
  Demux2 : Demux  Outputs=2
  Gain : Gain  Gain=1/Wbase
  Gain1 : Gain  Gain=1/Vbase
  Gain2 : Gain  Gain=Sbase/Vbase
  Gain3 : Gain  Gain=1/(Sbase/Vbase)
  MATLAB System1 : MATLABSystem  System=SimplusGT.Class.GridFormingVSI  Ts=Ts  Para=ApparatusPara  ApparatusType=ApparatusType  PowerFlow=PowerFlow  x0=x0  DiscreMethod=DiscreMethod  LinearizationTimes=LinearizationTimes  DirectFeedthrough=DirectFeedthrough  VirtualResistor=DiscreDampingFlag  EquiInitial=true  ElecPortIOs=[ 1, 2 ]  SimulateUsing=Code generation
      mask Type: SimplusGT.Class.GridFormingVSI
      mask Display:
      | disp('GridFormingVSI');
      | port_label('input',1,'u');
      | port_label('output',1,'y');
  Math Function2 : Math  Operator=mod  SignedPower=on
  Mux : Mux  Inputs=2
  Mux1 : Mux  Inputs=3
  Mux2 : Mux  Inputs=3
  Mux3 : Mux  Inputs=3
  PQ Calculation (dq-Frame) : Subsystem  AncestorBlock=|
      | SimplusGT/PQ Calculation
      | (dq-Frame)
      settings: LibrarySourceBlock=|
      | SimplusGT/PQ Calculation
      | (dq-Frame)
  R_VD : spsThreePhaseSeriesRLCBranchLib/Three-Phase Series RLC Branch  LConnTagsString=A|B|C  RConnTagsString=A|B|C  BranchType=R  Resistance=DiscreDampingValue*Vbase^2/Sbase  Inductance=1e-3  Capacitance=1e-6  Measurements=None
  "abc -> dq (Power-Invariant)" : Subsystem  AncestorBlock=|
      | SimplusGT/abc -> dq
      | (Power-Invariant)
      settings: LibrarySourceBlock=|
      | SimplusGT/abc -> dq
      | (Power-Invariant)
  "abc -> dq (Power-Invariant)1" : Subsystem  AncestorBlock=|
      | SimplusGT/abc -> dq
      | (Power-Invariant)
      settings: LibrarySourceBlock=|
      | SimplusGT/abc -> dq
      | (Power-Invariant)
  "dq -> abc (Power-Invariant)" : Subsystem  AncestorBlock=|
      | SimplusGT/dq -> abc
      | (Power-Invariant)
      settings: LibrarySourceBlock=|
      | SimplusGT/dq -> abc
      | (Power-Invariant)
  ia : spsControlledCurrentSourceLib/Controlled Current Source  Initialize=on  Source_Type=AC  Amplitude=0  Phase=0  Frequency=0  Measurements=None
  ia_m : spsCurrentMeasurementLib/Current Measurement  PhasorSimulation=off  OutputType=Complex  PSBequivalent=0
  ib : spsControlledCurrentSourceLib/Controlled Current Source  Initialize=on  Source_Type=AC  Amplitude=0  Phase=0  Frequency=0  Measurements=None
  ib_m : spsCurrentMeasurementLib/Current Measurement  PhasorSimulation=off  OutputType=Complex  PSBequivalent=0
  ic : spsControlledCurrentSourceLib/Controlled Current Source  Initialize=on  Source_Type=AC  Amplitude=0  Phase=0  Frequency=0  Measurements=None
  ic_m : spsCurrentMeasurementLib/Current Measurement  PhasorSimulation=off  OutputType=Complex  PSBequivalent=0
  va : spsVoltageMeasurementLib/Voltage Measurement  PhasorSimulation=off  OutputType=Complex  PSBequivalent=0
  vb : spsVoltageMeasurementLib/Voltage Measurement  PhasorSimulation=off  OutputType=Complex  PSBequivalent=0
  vc : spsVoltageMeasurementLib/Voltage Measurement  PhasorSimulation=off  OutputType=Complex  PSBequivalent=0
  a : PMIOPort  Side=Left
  b : PMIOPort  Port=2  Side=Left
  c : PMIOPort  Port=3  Side=Left
  n : PMIOPort  Port=4  Side=Left
  m : Outport
  wires:
  Demux/2 -> Mux/2
  Demux/1 -> Mux/1
  Mux/1 -> [i_dq]
  Demux/3 -> [w]
  Demux1/1 -> ia/1
  Demux1/2 -> ib/1
  va/1 -> Mux1/1
  vb/1 -> Mux1/2
  Mux1/1 -> Gain1/1
  [v_dq] -> Demux2/1
  Demux2/1 -> Mux2/1
  Demux2/2 -> Mux2/2
  [v_dq] -> Bus Creator/1  "v_dq"
  [i_dq_t] -> Bus Creator/2  "i_dq"
  [v_abc] -> Bus Creator/3  "v_abc"
  [i_abc_t] -> Bus Creator/4  "i_abc"
  [theta] -> Bus Creator/6  "theta"
  [v_abc] -> "abc -> dq (Power-Invariant)"/1(abc)
  [theta] -> "abc -> dq (Power-Invariant)"/2(theta)
  "abc -> dq (Power-Invariant)"/1(dq) -> [v_dq]
  [i_dq] -> "dq -> abc (Power-Invariant)"/1(dq)
  [theta] -> "dq -> abc (Power-Invariant)"/2(theta)
  "dq -> abc (Power-Invariant)"/1(abc) -> [i_abc]
  Mux2/1 -> MATLAB System1/1
  MATLAB System1/1 -> Demux/1
  vc/1 -> Mux1/3
  Demux1/3 -> ic/1
  Constant5/1 -> Math Function2/2
  Math Function2/1 -> [theta]
  Bus Creator/1 -> m/1
  [w] -> Gain/1  "w"
  Gain/1 -> Bus Creator/5  "w"
  [i_abc] -> Gain2/1
  [pq] -> Bus Creator/7  "pq"
  [v_dq] -> PQ Calculation (dq-Frame)/1(vdq)  "v_dq"
  [i_dq_t] -> PQ Calculation (dq-Frame)/2(idq)  "i_dq"
  PQ Calculation (dq-Frame)/1(pq) -> [pq]
  Gain2/1 -> Demux1/1
  Gain1/1 -> [v_abc]
  [v_dc] -> Bus Creator/8  "v_dc"
  Demux/4 -> Math Function2/1
  Constant/1 -> Mux2/3
  ic_m/1 -> Mux3/3
  ia_m/1 -> Mux3/1
  ib_m/1 -> Mux3/2
  Gain3/1 -> [i_abc_t]
  Mux3/1 -> Gain3/1
  [i_abc_t] -> "abc -> dq (Power-Invariant)1"/1(abc)
  [theta] -> "abc -> dq (Power-Invariant)1"/2(theta)
  "abc -> dq (Power-Invariant)1"/1(dq) -> [i_dq_t]
  connections:
  vb/LConn2 -- va/LConn2 -- vc/LConn2 -- R_VD/RConn3 -- R_VD/RConn2 -- R_VD/RConn1 -- ic/RConn1 -- ia/RConn1 -- ib/RConn1 -- n/RConn1
  R_VD/LConn1 -- va/LConn1 -- ia_m/RConn1 -- ia/LConn1
  R_VD/LConn2 -- ib_m/RConn1 -- vb/LConn1 -- ib/LConn1
  R_VD/LConn3 -- ic/LConn1 -- ic_m/RConn1 -- vc/LConn1
  ia_m/LConn1 -- a/RConn1
  ib_m/LConn1 -- b/RConn1
  ic_m/LConn1 -- c/RConn1

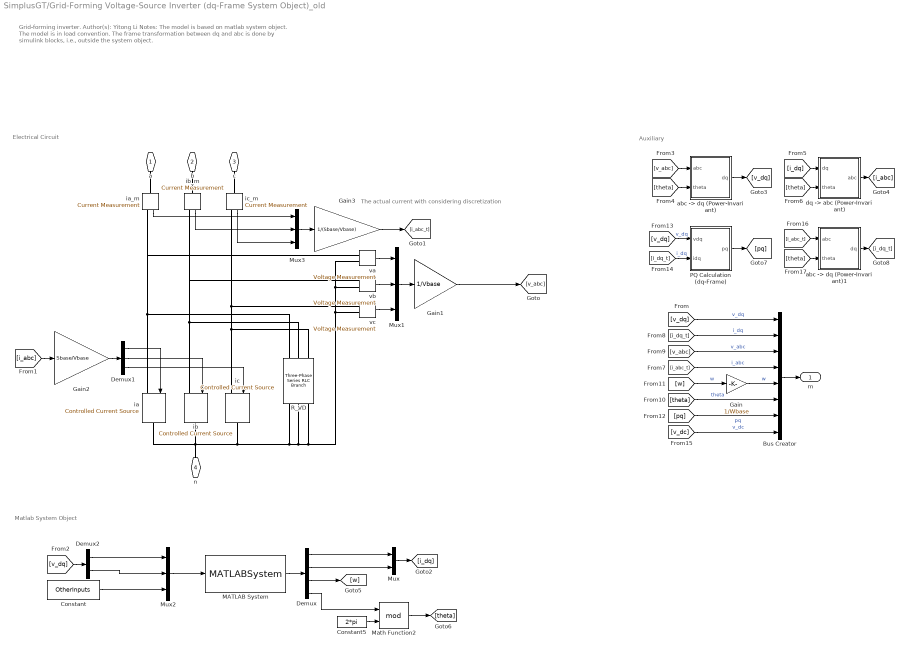
== system SimplusGT/Grid-Forming Voltage-Source Inverter (dq-Frame System Object)_old ==
  note: Matlab System Object
  note: Auxiliary
  note: Electrical Circuit
  note: Grid-forming inverter.
      |
      | Author(s): Yitong Li
      |
      | Notes:
      |
      | The model is based on matlab system object.
      |
      | The model is in load convention.
      |
      | The frame transformation between dq and abc is done by simulink blocks, i.e., outside the system object.
  note: The actual current with considering discretization
  Bus Creator : BusCreator  Inputs=8
  Constant : Constant  Value=OtherInputs
  Constant5 : Constant  Value=2*pi
  Demux : Demux
  Demux1 : Demux  Outputs=3
  Demux2 : Demux  Outputs=2
  Gain : Gain  Gain=1/Wbase
  Gain1 : Gain  Gain=1/Vbase
  Gain2 : Gain  Gain=Sbase/Vbase
  Gain3 : Gain  Gain=1/(Sbase/Vbase)
  MATLAB System : MATLABSystem  System=SimplusGT.Class.GridFormingVSI_old  Ts=Ts  Para=ApparatusPara  ApparatusType=ApparatusType  PowerFlow=PowerFlow  x0=x0  DiscreMethod=DiscreMethod  LinearizationTimes=LinearizationTimes  DirectFeedthrough=DirectFeedthrough  VirtualResistor=DiscreDampingFlag  EquiInitial=true  ElecPortIOs=[ 1, 2 ]  SimulateUsing=Code generation
      mask Type: SimplusGT.Class.GridFormingVSI_old
      mask Display:
      | disp('GridFormingVSI_old');
      | port_label('input',1,'u');
      | port_label('output',1,'y');
  Math Function2 : Math  Operator=mod  SignedPower=on
  Mux : Mux  Inputs=2
  Mux1 : Mux  Inputs=3
  Mux2 : Mux  Inputs=3
  Mux3 : Mux  Inputs=3
  PQ Calculation (dq-Frame) : Subsystem  AncestorBlock=|
      | SimplusGT/PQ Calculation
      | (dq-Frame)
      settings: LibrarySourceBlock=|
      | SimplusGT/PQ Calculation
      | (dq-Frame)
  R_VD : spsThreePhaseSeriesRLCBranchLib/Three-Phase Series RLC Branch  LConnTagsString=A|B|C  RConnTagsString=A|B|C  BranchType=R  Resistance=DiscreDampingValue*Vbase^2/Sbase  Inductance=1e-3  Capacitance=1e-6  Measurements=None
  "abc -> dq (Power-Invariant)" : Subsystem  AncestorBlock=|
      | SimplusGT/abc -> dq
      | (Power-Invariant)
      settings: LibrarySourceBlock=|
      | SimplusGT/abc -> dq
      | (Power-Invariant)
  "abc -> dq (Power-Invariant)1" : Subsystem  AncestorBlock=|
      | SimplusGT/abc -> dq
      | (Power-Invariant)
      settings: LibrarySourceBlock=|
      | SimplusGT/abc -> dq
      | (Power-Invariant)
  "dq -> abc (Power-Invariant)" : Subsystem  AncestorBlock=|
      | SimplusGT/dq -> abc
      | (Power-Invariant)
      settings: LibrarySourceBlock=|
      | SimplusGT/dq -> abc
      | (Power-Invariant)
  ia : spsControlledCurrentSourceLib/Controlled Current Source  Initialize=on  Source_Type=AC  Amplitude=0  Phase=0  Frequency=0  Measurements=None
  ia_m : spsCurrentMeasurementLib/Current Measurement  PhasorSimulation=off  OutputType=Complex  PSBequivalent=0
  ib : spsControlledCurrentSourceLib/Controlled Current Source  Initialize=on  Source_Type=AC  Amplitude=0  Phase=0  Frequency=0  Measurements=None
  ib_m : spsCurrentMeasurementLib/Current Measurement  PhasorSimulation=off  OutputType=Complex  PSBequivalent=0
  ic : spsControlledCurrentSourceLib/Controlled Current Source  Initialize=on  Source_Type=AC  Amplitude=0  Phase=0  Frequency=0  Measurements=None
  ic_m : spsCurrentMeasurementLib/Current Measurement  PhasorSimulation=off  OutputType=Complex  PSBequivalent=0
  va : spsVoltageMeasurementLib/Voltage Measurement  PhasorSimulation=off  OutputType=Complex  PSBequivalent=0
  vb : spsVoltageMeasurementLib/Voltage Measurement  PhasorSimulation=off  OutputType=Complex  PSBequivalent=0
  vc : spsVoltageMeasurementLib/Voltage Measurement  PhasorSimulation=off  OutputType=Complex  PSBequivalent=0
  a : PMIOPort  Side=Left
  b : PMIOPort  Port=2  Side=Left
  c : PMIOPort  Port=3  Side=Left
  n : PMIOPort  Port=4  Side=Left
  m : Outport
  wires:
  Demux/2 -> Mux/2
  Demux/1 -> Mux/1
  Mux/1 -> [i_dq]
  Demux/3 -> [w]
  Demux1/1 -> ia/1
  Demux1/2 -> ib/1
  va/1 -> Mux1/1
  vb/1 -> Mux1/2
  Mux1/1 -> Gain1/1
  [v_dq] -> Demux2/1
  Demux2/1 -> Mux2/1
  Demux2/2 -> Mux2/2
  [v_dq] -> Bus Creator/1  "v_dq"
  [i_dq_t] -> Bus Creator/2  "i_dq"
  [v_abc] -> Bus Creator/3  "v_abc"
  [i_abc_t] -> Bus Creator/4  "i_abc"
  [theta] -> Bus Creator/6  "theta"
  [v_abc] -> "abc -> dq (Power-Invariant)"/1(abc)
  [theta] -> "abc -> dq (Power-Invariant)"/2(theta)
  "abc -> dq (Power-Invariant)"/1(dq) -> [v_dq]
  [i_dq] -> "dq -> abc (Power-Invariant)"/1(dq)
  [theta] -> "dq -> abc (Power-Invariant)"/2(theta)
  "dq -> abc (Power-Invariant)"/1(abc) -> [i_abc]
  Mux2/1 -> MATLAB System/1
  MATLAB System/1 -> Demux/1
  vc/1 -> Mux1/3
  Demux1/3 -> ic/1
  Constant5/1 -> Math Function2/2
  Math Function2/1 -> [theta]
  Bus Creator/1 -> m/1
  [w] -> Gain/1  "w"
  Gain/1 -> Bus Creator/5  "w"
  [i_abc] -> Gain2/1
  [pq] -> Bus Creator/7  "pq"
  [v_dq] -> PQ Calculation (dq-Frame)/1(vdq)  "v_dq"
  [i_dq_t] -> PQ Calculation (dq-Frame)/2(idq)  "i_dq"
  PQ Calculation (dq-Frame)/1(pq) -> [pq]
  Gain2/1 -> Demux1/1
  Gain1/1 -> [v_abc]
  [v_dc] -> Bus Creator/8  "v_dc"
  Demux/4 -> Math Function2/1
  Constant/1 -> Mux2/3
  ic_m/1 -> Mux3/3
  ia_m/1 -> Mux3/1
  ib_m/1 -> Mux3/2
  Gain3/1 -> [i_abc_t]
  Mux3/1 -> Gain3/1
  [i_abc_t] -> "abc -> dq (Power-Invariant)1"/1(abc)
  [theta] -> "abc -> dq (Power-Invariant)1"/2(theta)
  "abc -> dq (Power-Invariant)1"/1(dq) -> [i_dq_t]
  connections:
  vb/LConn2 -- va/LConn2 -- vc/LConn2 -- R_VD/RConn3 -- R_VD/RConn2 -- R_VD/RConn1 -- ic/RConn1 -- ia/RConn1 -- ib/RConn1 -- n/RConn1
  R_VD/LConn1 -- va/LConn1 -- ia_m/RConn1 -- ia/LConn1
  R_VD/LConn2 -- ib_m/RConn1 -- vb/LConn1 -- ib/LConn1
  R_VD/LConn3 -- ic/LConn1 -- ic_m/RConn1 -- vc/LConn1
  ia_m/LConn1 -- a/RConn1
  ib_m/LConn1 -- b/RConn1
  ic_m/LConn1 -- c/RConn1
